simulink library "marine_hydro"  (Simulink 7.4)
settings: Solver=ode45  SolverMode=SingleTasking  StartTime=0.0  StopTime=10.0  RelTol=1e-3
undefined symbols (not defined in the file or in its folder): Hoerner, magnitude, slcm, vessel, vesselABC
libraries: simulink x60, marine_gnc x22, marine_hydro x9
(part 3 of 4)

== system marine_hydro/Hydro Library/Wave loads (U=0)/psi1 ==
  k : Inport  OutDataType=sfix(16)  OutScaling=2^0
  0 or 1 : Inport  Port=2  OutDataType=sfix(16)  OutScaling=2^0
  Gain1 : Gain  Gain=20  ParameterDataType=sfix(16)  ParameterScaling=2^0  OutDataType=sfix(16)  OutScaling=2^0
  Gain2 : Gain  Gain=10  ParameterDataType=sfix(16)  ParameterScaling=2^0  OutDataType=sfix(16)  OutScaling=2^0
  Product : Product  OutDataType=sfix(16)  OutScaling=2^0  RndMeth=Zero
  Sum7 : Sum  Inputs=-+|  OutDataType=sfix(16)  OutScaling=2^0
  Sum8 : Sum  Inputs=++|  OutDataType=sfix(16)  OutScaling=2^0
  const : Constant  Value=18  OutDataType=sfix(16)  OutScaling=2^0
  psi : Outport  OutDataType=sfix(16)  OutScaling=2^0
  wires:
  const/1 -> Sum7/2
  Sum7/1 -> Gain1/1
  Gain1/1 -> Product/1
  Product/1 -> Sum8/2
  Gain2/1 -> Sum8/1
  k/1 -> Sum7/1, Gain2/1
  Sum8/1 -> psi/1
  0 or 1/1 -> Product/2

== system marine_hydro/Hydro Library/Wave loads (U=0)/psi2 ==
  k : Inport  OutDataType=sfix(16)  OutScaling=2^0
  0 or 1 : Inport  Port=2  OutDataType=sfix(16)  OutScaling=2^0
  Gain1 : Gain  Gain=20  ParameterDataType=sfix(16)  ParameterScaling=2^0  OutDataType=sfix(16)  OutScaling=2^0
  Gain2 : Gain  Gain=10  ParameterDataType=sfix(16)  ParameterScaling=2^0  OutDataType=sfix(16)  OutScaling=2^0
  Product : Product  OutDataType=sfix(16)  OutScaling=2^0  RndMeth=Zero
  Sum7 : Sum  Inputs=-+|  OutDataType=sfix(16)  OutScaling=2^0
  Sum8 : Sum  Inputs=++|  OutDataType=sfix(16)  OutScaling=2^0
  const : Constant  Value=18  OutDataType=sfix(16)  OutScaling=2^0
  psi : Outport  OutDataType=sfix(16)  OutScaling=2^0
  wires:
  const/1 -> Sum7/2
  Sum7/1 -> Gain1/1
  Gain1/1 -> Product/1
  Product/1 -> Sum8/2
  Gain2/1 -> Sum8/1
  k/1 -> Sum7/1, Gain2/1
  Sum8/1 -> psi/1
  0 or 1/1 -> Product/2

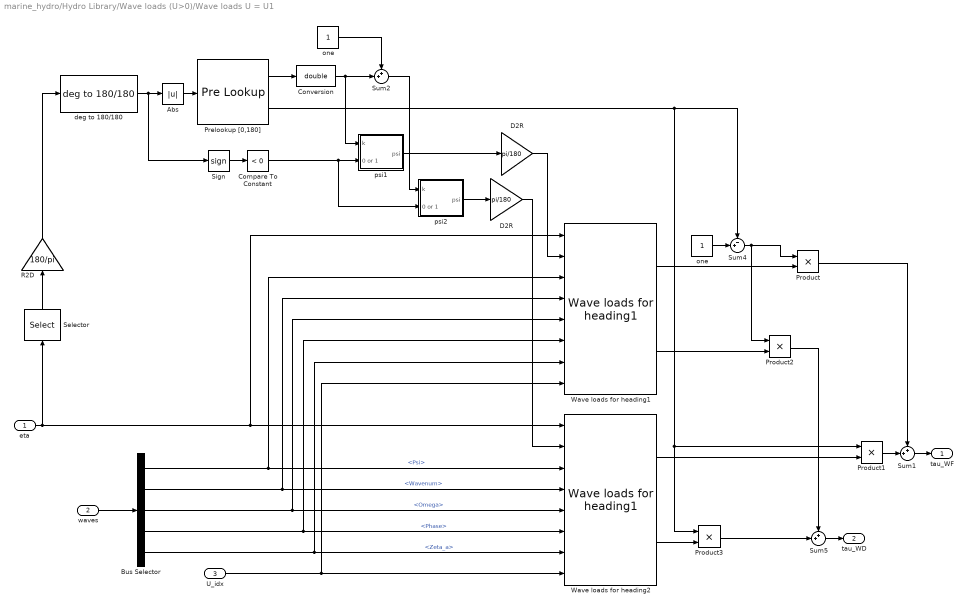
== system marine_hydro/Hydro Library/Wave loads (U>0)/Wave loads U = U1 ==
  eta : Inport  OutDataType=sfix(16)  OutScaling=2^0
  waves : Inport  Port=2  OutDataType=sfix(16)  OutScaling=2^0
  U_idx : Inport  Port=3  OutDataType=sfix(16)  OutScaling=2^0
  Abs : Abs  SaturateOnIntegerOverflow=on
  Bus Selector : BusSelector  OutputSignals=Psi,Wavenum,Omega,Phase,Zeta_a
  Compare To Constant : simulink/Logic and Bit Operations/Compare To Constant  SystemSampleTime=-1  relop=<  const=0  LogicOutDataTypeMode=uint8  ZeroCross=off
  Conversion : DataTypeConversion  OutDataTypeMode=double  OutDataType=sfix(16)  OutScaling=2^0  OutDataTypeStr=double
  D2R : Gain  Gain=pi/180  ParameterDataType=sfix(16)  ParameterScaling=2^0  OutDataType=sfix(16)  OutScaling=2^0
  "D2R " : Gain  Gain=pi/180  ParameterDataType=sfix(16)  ParameterScaling=2^0  OutDataType=sfix(16)  OutScaling=2^0
  Prelookup [0,180] : PreLookup  BreakpointsData=[0:10:180]  IndexSearchMethod=Evenly spaced points  BeginIndexSearchUsingPreviousIndexResult=on  IndexDataType=sfix(16)  FractionDataType=sfix(16)  FractionScaling=2^0
  Product{,1..3} (4 alike) : Product  OutDataType=sfix(16)  OutScaling=2^0  RndMeth=Zero
  R2D : Gain  Gain=180/pi  ParameterDataType=sfix(16)  ParameterScaling=2^0  OutDataType=sfix(16)  OutScaling=2^0
  Selector : Selector  InputPortWidth=6  IndexOptions=Index vector (dialog)  Indices=[6]  OutputSizes=1
  Sign : Signum
  Sum1 : Sum  Inputs=++|  OutDataType=sfix(16)  OutScaling=2^0
  Sum2 : Sum  Inputs=++|  OutDataType=sfix(16)  OutScaling=2^0
  Sum4 : Sum  Inputs=-+|  OutDataType=sfix(16)  OutScaling=2^0
  Sum5 : Sum  Inputs=++|  OutDataType=sfix(16)  OutScaling=2^0
  Wave loads for heading1 : marine_hydro/Hydro Library/Wave loads for heading1  SystemSampleTime=-1  ForceRAO_Freq=vessel.forceRAO.w  WD_Freq=vessel.driftfrc.w  RAO_Vel=vessel.velocities  ForceRAO_Amp=vessel.forceRAO.amp  ForceRAO_Phase=vessel.forceRAO.phase  WD_Amp=vessel.driftfrc.amp  RAO_add_omega_0=on  RAO_add_omega_inf=on
  Wave loads for heading2 : marine_hydro/Hydro Library/Wave loads for heading1  SystemSampleTime=-1  ForceRAO_Freq=vessel.forceRAO.w  WD_Freq=vessel.driftfrc.w  RAO_Vel=vessel.velocities  ForceRAO_Amp=vessel.forceRAO.amp  ForceRAO_Phase=vessel.forceRAO.phase  WD_Amp=vessel.driftfrc.amp  RAO_add_omega_0=on  RAO_add_omega_inf=on
  deg to 180/180 : marine_gnc/Utilities/Math Operations/deg to 180//180  SystemSampleTime=-1
  one : Constant  OutDataType=sfix(16)  OutScaling=2^0
  "one " : Constant  OutDataType=sfix(16)  OutScaling=2^0
  psi1 : Subsystem
  psi2 : Subsystem
  tau_WF : Outport  OutDataType=sfix(16)  OutScaling=2^0
  tau_WD : Outport  Port=2  OutDataType=sfix(16)  OutScaling=2^0
  wires:
  R2D/1 -> deg to 180/180/1
  Selector/1 -> R2D/1
  Sum5/1 -> tau_WD/1
  waves/1 -> Bus Selector/1
  Sum1/1 -> tau_WF/1
  "D2R "/1 -> Wave loads for heading2/2
  D2R/1 -> Wave loads for heading1/2
  psi2/1(psi) -> "D2R "/1
  Conversion/1 -> psi1/1(k), Sum2/2
  Prelookup [0,180]/2 -> Sum4/1, Product1/1, Product3/1
  psi1/1(psi) -> D2R/1
  Compare To Constant/1 -> psi2/2(0 or 1), psi1/2(0 or 1)
  Sign/1 -> Compare To Constant/1
  Abs/1 -> Prelookup [0,180]/1
  deg to 180/180/1 -> Sign/1, Abs/1
  Sum2/1 -> psi2/1(k)
  one/1 -> Sum2/1
  Prelookup [0,180]/1 -> Conversion/1
  Product2/1 -> Sum5/1
  Product3/1 -> Sum5/2
  Wave loads for heading1/2 -> Product2/2
  Sum4/1 -> Product2/1, Product/1
  "one "/1 -> Sum4/2
  Product1/1 -> Sum1/2
  Product/1 -> Sum1/1
  Wave loads for heading1/1 -> Product/2
  Bus Selector/5 -> Wave loads for heading1/7, Wave loads for heading2/7  "<Zeta_a>"
  Bus Selector/4 -> Wave loads for heading1/6, Wave loads for heading2/6  "<Phase>"
  Bus Selector/3 -> Wave loads for heading1/5, Wave loads for heading2/5  "<Omega>"
  Bus Selector/2 -> Wave loads for heading1/4, Wave loads for heading2/4  "<Wavenum>"
  Bus Selector/1 -> Wave loads for heading1/3, Wave loads for heading2/3  "<Psi>"
  eta/1 -> Selector/1, Wave loads for heading1/1, Wave loads for heading2/1
  Wave loads for heading2/2 -> Product3/2
  Wave loads for heading2/1 -> Product1/2
  U_idx/1 -> Wave loads for heading1/8, Wave loads for heading2/8

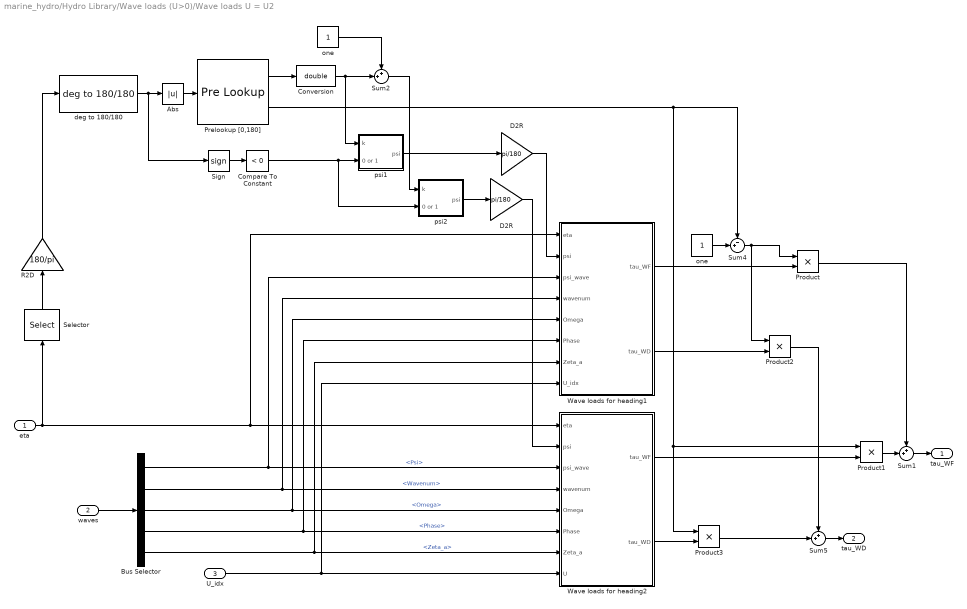
== system marine_hydro/Hydro Library/Wave loads (U>0)/Wave loads U = U2 ==
  eta : Inport  OutDataType=sfix(16)  OutScaling=2^0
  waves : Inport  Port=2  OutDataType=sfix(16)  OutScaling=2^0
  U_idx : Inport  Port=3  OutDataType=sfix(16)  OutScaling=2^0
  Abs : Abs  SaturateOnIntegerOverflow=on
  Bus Selector : BusSelector  OutputSignals=Psi,Wavenum,Omega,Phase,Zeta_a
  Compare To Constant : simulink/Logic and Bit Operations/Compare To Constant  SystemSampleTime=-1  relop=<  const=0  LogicOutDataTypeMode=uint8  ZeroCross=off
  Conversion : DataTypeConversion  OutDataTypeMode=double  OutDataType=sfix(16)  OutScaling=2^0  OutDataTypeStr=double
  D2R : Gain  Gain=pi/180  ParameterDataType=sfix(16)  ParameterScaling=2^0  OutDataType=sfix(16)  OutScaling=2^0
  "D2R " : Gain  Gain=pi/180  ParameterDataType=sfix(16)  ParameterScaling=2^0  OutDataType=sfix(16)  OutScaling=2^0
  Prelookup [0,180] : PreLookup  BreakpointsData=[0:10:180]  IndexSearchMethod=Evenly spaced points  BeginIndexSearchUsingPreviousIndexResult=on  IndexDataType=sfix(16)  FractionDataType=sfix(16)  FractionScaling=2^0
  Product{,1..3} (4 alike) : Product  OutDataType=sfix(16)  OutScaling=2^0  RndMeth=Zero
  R2D : Gain  Gain=180/pi  ParameterDataType=sfix(16)  ParameterScaling=2^0  OutDataType=sfix(16)  OutScaling=2^0
  Selector : Selector  InputPortWidth=6  IndexOptions=Index vector (dialog)  Indices=[6]  OutputSizes=1
  Sign : Signum
  Sum1 : Sum  Inputs=++|  OutDataType=sfix(16)  OutScaling=2^0
  Sum2 : Sum  Inputs=++|  OutDataType=sfix(16)  OutScaling=2^0
  Sum4 : Sum  Inputs=-+|  OutDataType=sfix(16)  OutScaling=2^0
  Sum5 : Sum  Inputs=++|  OutDataType=sfix(16)  OutScaling=2^0
  Wave loads for heading1 : Subsystem  AncestorBlock=marine_gnc/Models/Environmental Loads/Force RAO  mask(Force RAO){ForceRAO_Freq=vessel.forceRAO.w, WD_Freq=vessel.driftfrc.w, RAO_Vel=vessel.velocities, ForceRAO_Amp=vessel.forceRAO.amp, ForceRAO_Phase=vessel.forceRAO.phase, WD_Amp=vessel.driftfrc.amp, RAO_add_omega_0=on, RAO_add_omega_inf=on}
      mask prompts: ForceRAO_Freq "Vector of frequencies ForceRAO_Freq (rad/s)"; WD_Freq "Vector of frequencies WD_Freq (rad/s)"; RAO_Vel "Vector of velocities RAO_Vel (m/s)"; ForceRAO_Amp "6DOF Cell array with tables of Amplitudes ForceRAO_Amp"; ForceRAO_Phase "6DOF Cell array with tables of Phases ForceRAO_Phase (rad)"; WD_Amp "6DOF Cell array with tables of Amplitudes WD_Amp"; RAO_add_omega_0 "Add asymptotic RAO values for omega = 0"; RAO_add_omega_inf "Add asymptotic RAO values for omega = inf"
      mask help:
      | Calculate the 6 degrees-of-freedom (DOF) wave-frequency excitation forces tau_WF for a vessel from its Force Response Amplitude Operators (Force RAOs) and a sea state defined by a set of harmonic waves. The block takes the "Waves" bus from the MSS Waves block as input, as well as the vessel low-frequency (LF) motion in terms of the generalized position vector eta and mean surge velocity U. See help for details.
      |
      | Authors: Oyvind N. Smogeli and Thor I. Fossen, 2005-05-03
      mask init:
      | % use only nonzero increasing velocities, if zero element add eps
      | Nvel = length(RAO_Vel);
      | 
      | if Nvel == 1
      |     RAO_Vel = [0 1e10];   % use one data set for U=0 and one dummy set for u=1e10
      |     Nvel = 2;
      | end
      | 
      | for dof = 1:6
      |     TempFA{dof}  = ForceRAO_Amp{dof}(:,:,1:Nvel);
      |     TempFP{dof}  = ForceRAO_Phase{dof}(:,:,1:Nvel);
      | end
      | 
      | for dof = 1:3
      |     TempWA{dof}  = WD_Amp{dof}(:,:,1:Nvel);
      | end
      | 
      | clear ForceRAO_Amp ForceRAO_Phase WD_Amp WD_Phase
      | 
      | ForceRAO_Amp   = TempFA;
      | ForceRAO_Phase = TempFP;
      | WD_Amp         = TempWA;
      | 
      | % Add RAO values for zero frequency: use values for lowest given frequency
      | if RAO_add_omega_0 > 0
      | 	
      | 	if min(ForceRAO_Freq) > 0
      | 				
      | 		ForceRAO_Freq = [0 ForceRAO_Freq];
      | 		for dofno = 1:6
      | 			ForceRAO_Amp{dofno}   = [ForceRAO_Amp{dofno}(1,:,:);   ForceRAO_Amp{dofno}];
      | 			ForceRAO_Phase{dofno} = [ForceRAO_Phase{dofno}(1,:,:); ForceRAO_Phase{dofno}];
      |         end
      | 
      |     end
      |     
      | 	if min(WD_Freq) > 0
      |         
      | 		WD_Freq = [0 WD_Freq];
      | 		for dofno = 1:3
      | 			WD_Amp{dofno} = [WD_Amp{dofno}(1,:,:); WD_Amp{dofno}];
      | 		end        
      |         
      | 	end
      | 	
      | end
      | 
      | % Add RAO values for high frequency: use values for highest given frequency
      | maxfreq = 10;
      | if RAO_add_omega_inf > 0
      | 
      | 	if max(ForceRAO_Freq) < maxfreq
      | 			
      | 		newfreq = 2*max(ForceRAO_Freq) - ForceRAO_Freq(length(ForceRAO_Freq)-1);
      | 		
      | 		ForceRAO_Freq = [ForceRAO_Freq newfreq maxfreq];
      | 		for dofno = 1:6
      | 			ForceRAO_Amp{dofno}   = [ForceRAO_Amp{dofno};   zeros(2, 36, Nvel)];
      | 			ForceRAO_Phase{dofno} = [ForceRAO_Phase{dofno}; zeros(2, 36, Nvel)];
      | 		end
      | 		
      |     end
      | 
      | 	if max(WD_Freq) < maxfreq
      | 			
      | 		newfreq = 2*max(WD_Freq) - WD_Freq(length(WD_Freq)-1);
      | 		
      | 		WD_Freq = [WD_Freq newfreq maxfreq];
      | 		for dofno = 1:3
      | 			WD_Amp{dofno} = [WD_Amp{dofno}; zeros(2, 36, Nvel)];
      | 		end
      | 		
      |     end
      |     
      | end
      mask Help:
      | <b>Part of the Marine Systems Simulator: MSS</b><br>
      | <br>
      | Calculate the 6 degrees-of-freedom (DOF) wave-frequency excitation forces tau_WF
      | for a vessel from its Force Response Amplitude Operators (Force RAOs) and a sea
      | state defined by a set of harmonic waves. The block takes the &quot;Waves&quot; bus from
      | the MSS Waves block as input, as well as the vessel low-frequency (LF) motion in
      | terms of the generalized position vector eta and mean surge velocity U.<p>The Force RAOs are defined in terms of a
      | vector of frequencies (RAO_Freq), a vector of directions (RAO_Dir), a vector of
      | velocities (RAO_Dir), a 6DOF cell array of 3D matrices with amplitudes
      | (RAO_Amp), and a 6DOF cell array of 3D matrices with phases (RAO_Phase), which
      | are all input in the block mask. The first dimension of the 3D matrices
      | corresponds to the frequencies, the second to the directions, and the third to
      | the velocities, such that e.g. the amplitude amp in heave (DOF #3) for frequency
      | number n_f, direction number n_d and velocity number n_v can be found from a =
      | RAO_Amp{3}(n_f, n_d, n_v).</p>
      | <p><b>Inputs:</b></p>
      | <p>Waves:&nbsp;&nbsp;&nbsp;&nbsp;&nbsp;&nbsp;&nbsp;&nbsp;&nbsp;&nbsp;&nbsp; Bus
      | containing the following signals<br>
      | &nbsp;&nbsp;&nbsp; Zeta_a:&nbsp;&nbsp;&nbsp;&nbsp;&nbsp;&nbsp;&nbsp; Vector of harmonic wave amplitudes [m]<br>
      | &nbsp;&nbsp;&nbsp; Omega:&nbsp;&nbsp;&nbsp;&nbsp;&nbsp;&nbsp; Vector of harmonic wave frequencies [rad/s]<br>
      | &nbsp;&nbsp;&nbsp; Phase:&nbsp;&nbsp;&nbsp;&nbsp;&nbsp;&nbsp;&nbsp;&nbsp; Vector of harmonic wave phases (random) [rad]<br>
      | &nbsp;&nbsp;&nbsp; Wavenum:&nbsp;&nbsp;&nbsp; Vector of harmonic wave numbers [1/m]<br>
      | &nbsp;&nbsp;&nbsp; Psi:&nbsp;&nbsp;&nbsp;&nbsp;&nbsp;&nbsp;&nbsp;&nbsp;&nbsp;&nbsp;&nbsp;&nbsp;&nbsp; Vector of harmonic wave directions [rad]</p>
      | <p>eta_LF:&nbsp;&nbsp;&nbsp;&nbsp;&nbsp;&nbsp;&nbsp;&nbsp;&nbsp;&nbsp;&nbsp;
      | Generalized 6DOF n-frame low-frequency position vector [x (m), y (m), z (m),
      | theta (rad), phi (rad), psi (rad)]<br>
      | U:&nbsp;&nbsp;&nbsp;&nbsp;&nbsp;&nbsp;&nbsp;&nbsp;&nbsp;&nbsp;&nbsp;&nbsp;&nbsp;&nbsp;&nbsp;&nbsp;&nbsp;&nbsp;&nbsp;
      | Low-frequency (mean) surge velocity&nbsp; [m/s]</p>
      | <p><b>Outputs:</b></p>
      | <p>tau_WF:&nbsp;&nbsp;&nbsp;&nbsp;&nbsp;&nbsp;&nbsp;&nbsp;&nbsp; Generalized
      | 6DOF h-frame force vector [X (N), Y (N), Z (N), K (Nm), M (Nm), N (Nm)]</p>
      | <p><b>Model validity:</b></p>
      | <p>The validity of the block is dependent on the validity of the given
      | RAO data set.</p>
      | <p>A proper RAO to be used with this block should contain at least 1 velocity, 5
      | directions (e.g. 0, 45, 90, 135 and 180 degrees) and 10-20 frequencies, for all
      | 6 DOF (surge, sway, heave, roll, pitch, yaw).</p>
      | <p>The block performs linear interpolation in frequencies and directions, and
      | uses the data set for the velocity closest to the input velocity (i.e. 'nearest'
      | interpolation in velocity). If the block recieves an input wave frequency or relative
      | wave direction outside the span of the data vectors RAO_Freq or RAO_Dir
      | respectively, the simulation stops and an error is returned. This means that a well-defined
      | RAO must contain data for both 0 and 180 degrees, and for frequencies covering
      | the desired range of wave frequencies. If desired, asymptotic values can be
      | automatically added for zero and infinity frequency to avoid runtime errors if
      | the wave freqeuncy exceeds the values in RAO_Freq (see checkboxes in the mask). </p>
      | <p>IMPORTANT NOTE: The RAO theory upon which this block is based is in reality
      | only valid when the vessel low-frequency (h-frame) motion is a constant surge
      | velocity only, and the vessel is performing wave-frequency oscillations about
      | the steadily translating h-frame.This means that the outputs from the block when
      | manoeuvering -- i.e. changing the surge velocity and/or yaw angle -- must be
      | interpreted with some care. A jump in the output must be expected when changing
      | between two velocity data sets, and frequency warping expected when changing the
      | yaw angle (due to interpolation in the phase). It is therefore recommended to
      | use backlash on the input velocity to avoid transient switching, and a quantized
      | yaw angle with backlash. The latter will lead to jump in the ouput when the yaw
      | angle changes from one quantized value to another, but will give better results
      | when keeping within one quantizer interval. The quantized yaw angle with
      | backlash and velocity with backlash are available as options via checkboxes in
      | the mask. If either of these are activated, proper values for the yaw
      | quantization interval, yaw backlash width, and the the speed backlash width
      | respectively must be set. Typical values could be a yaw quantization interval of
      | 5 degrees, yaw backlash width of 1/4-1/5 of the quantization interval, and speed
      | backlash width of 1 m/s. To avoid the most rapid transients when switching
      | between data sets, output smoothing is available as an option in the mask. If
      | this is enabled, the output during a transent is rate limited according to the
      | fastest recorded signal rate during normal operation.</p>
      | <p><b>Example mask input:</b></p><p>
      | As an example, the format of the mask input for 2 velocities, 3 directions and 5
      | frequencies is as follows:<p>RAO_Freq = [f1 f2 f3 f4 f5]<br>
      | RAO_Dir = [d1 d2 d3]<br>
      | RAO_Vel = [v1 v2]<p>Surge:<br>
      | RAO_Amp{1}(:,:,1)&nbsp; = [a1_111 a1_121 a1_131; a1_211 a1_221 a1_231; a1_311
      | a1_321 a1_331; a1_411 a1_421 a1_431; a1_511 a1_521 a1_531]<br>
      | RAO_Amp{1}(:,:,2)&nbsp; = [a1_112 a1_122 a1_132; a1_212 a1_222 a1_232; a1_312
      | a1_322 a1_332; a1_412 a1_422 a1_432; a1_512 a1_522 a1_532]<br>
      | RAO_Phase{1}(:,:,1) = [p1_111 p1_121 p1_131; p1_211 p1_221 p1_231; p1_311 p1_321
      | p1_331; p1_411 p1_421 p1_431; p1_511 p1_521 p1_531]<br>
      | RAO_Phase{1}(:,:,2) = [p1_112 p1_122 p1_132; p1_212 p1_222 p1_232; p1_312 p1_322
      | p1_332; p1_412 p1_422 p1_432; p1_512 p1_522 p1_532]<p>Sway:<br>
      | RAO_Amp{2}(:,:,1)&nbsp; = [a2_111 a2_121 a2_131; a2_211 a2_221 a2_231; a2_311
      | a2_321 a2_331; a2_411 a2_421 a2_431; a2_511 a2_521 a2_531]<br>
      | RAO_Amp{2}(:,:,2)&nbsp; = [a2_112 a2_122 a2_132; a2_212 a2_222 a2_232; a2_312
      | a2_322 a2_332; a2_412 a2_422 a2_432; a2_512 a2_522 a2_532]<br>
      | RAO_Phase{2}(:,:,1) = [p2_111 p2_121 p2_131; p2_211 p2_221 p2_231; p2_311 p2_321
      | p2_331; p2_411 p2_421 p2_431; p2_511 p2_521 p2_531]<br>
      | RAO_Phase{2}(:,:,2) = [p2_112 p2_122 p2_132; p2_212 p2_222 p2_232; p2_312 p2_322
      | p2_332; p2_412 p2_422 p2_432; p2_512 p2_522 p2_532]<p>...<p>Yaw:<br>
      | RAO_Amp{6}(:,:,1)&nbsp; = [a6_111 a6_121 a6_131; a6_211 a6_221 a6_231; a6_311
      | a6_321 a6_331; a6_411 a6_421 a6_431; a6_511 a6_521 a6_531]<br>
      | RAO_Amp{6}(:,:,2)&nbsp; = [a6_112 a6_122 a6_132; a6_212 a6_222 a6_232; a6_312
      | a6_322 a6_332; a6_412 a6_422 a6_432; a6_512 a6_522 a6_532]<br>
      | RAO_Phase{6}(:,:,1) = [p6_111 p6_121 p6_131; p6_211 p6_221 p6_231; p6_311 p6_321
      | p6_331; p6_411 p6_421 p6_431; p6_511 p6_521 p6_531]<br>
      | RAO_Phase{6}(:,:,2) = [p6_112 p6_122 p6_132; p6_212 p6_222 p6_232; p6_312 p6_322
      | p6_332; p6_412 p6_422 p6_432; p6_512 p6_522 p6_532]<p>where now for example the
      | amplitude and phase in sway (DOF 2) for frequency f5, direction d3 and velocity
      | v1 are given by RAO_Amp{2}(5,3,1) = a2_531 and RAO_Phase{2}(5,3,1) = p2_531.<p>
      | <b>Copyright (C) NTNU 2005</b></p>
      | <p><b>Author:</b> Oyvind N. Smogeli, 2005-05-03</p>
  Wave loads for heading2 : Subsystem  AncestorBlock=marine_gnc/Models/Environmental Loads/Force RAO  mask(Force RAO){ForceRAO_Freq=vessel.forceRAO.w, WD_Freq=vessel.driftfrc.w, RAO_Vel=vessel.velocities, ForceRAO_Amp=vessel.forceRAO.amp, ForceRAO_Phase=vessel.forceRAO.phase, WD_Amp=vessel.driftfrc.amp, RAO_add_omega_0=on, RAO_add_omega_inf=on}
      mask prompts: ForceRAO_Freq "Vector of frequencies ForceRAO_Freq (rad/s)"; WD_Freq "Vector of frequencies WD_Freq (rad/s)"; RAO_Vel "Vector of velocities RAO_Vel (m/s)"; ForceRAO_Amp "6DOF Cell array with tables of Amplitudes ForceRAO_Amp"; ForceRAO_Phase "6DOF Cell array with tables of Phases ForceRAO_Phase (rad)"; WD_Amp "6DOF Cell array with tables of Amplitudes WD_Amp"; RAO_add_omega_0 "Add asymptotic RAO values for omega = 0"; RAO_add_omega_inf "Add asymptotic RAO values for omega = inf"
      mask help:
      | Calculate the 6 degrees-of-freedom (DOF) wave-frequency excitation forces Tau_WF for a vessel from its Force Response Amplitude Operators (Force RAOs) and a sea state defined by a set of harmonic waves. The block takes the "Waves" bus from the MSS Waves block as input, as well as the vessel low-frequency (LF) motion in terms of the generalized position vector eta_LF and mean surge velocity U. See help for details.
      |
      | Copyright (C) NTNU 2005
      | Author: Oyvind N. Smogeli, 2005-05-03
      mask init: same as marine_hydro/Hydro Library/Wave loads (U>0)/Wave loads U = U2/Wave loads for heading1
      mask Help:
      | <b>Part of the Marine Systems Simulator: MSS</b><br>
      | <br>
      | Calculate the 6 degrees-of-freedom (DOF) wave-frequency excitation forces Tau_WF
      | for a vessel from its Force Response Amplitude Operators (Force RAOs) and a sea
      | state defined by a set of harmonic waves. The block takes the &quot;Waves&quot; bus from
      | the MSS Waves block as input, as well as the vessel low-frequency (LF) motion in
      | terms of the generalized position vector eta_LF and mean surge velocity U.<p>The Force RAOs are defined in terms of a
      | vector of frequencies (RAO_Freq), a vector of directions (RAO_Dir), a vector of
      | velocities (RAO_Dir), a 6DOF cell array of 3D matrices with amplitudes
      | (RAO_Amp), and a 6DOF cell array of 3D matrices with phases (RAO_Phase), which
      | are all input in the block mask. The first dimension of the 3D matrices
      | corresponds to the frequencies, the second to the directions, and the third to
      | the velocities, such that e.g. the amplitude amp in heave (DOF #3) for frequency
      | number n_f, direction number n_d and velocity number n_v can be found from a =
      | RAO_Amp{3}(n_f, n_d, n_v).</p>
      | <p><b>Inputs:</b></p>
      | <p>Waves:&nbsp;&nbsp;&nbsp;&nbsp;&nbsp;&nbsp;&nbsp;&nbsp;&nbsp;&nbsp;&nbsp; Bus
      | containing the following signals<br>
      | &nbsp;&nbsp;&nbsp; Zeta_a:&nbsp;&nbsp;&nbsp;&nbsp;&nbsp;&nbsp;&nbsp; Vector of harmonic wave amplitudes [m]<br>
      | &nbsp;&nbsp;&nbsp; Omega:&nbsp;&nbsp;&nbsp;&nbsp;&nbsp;&nbsp; Vector of harmonic wave frequencies [rad/s]<br>
      | &nbsp;&nbsp;&nbsp; Phase:&nbsp;&nbsp;&nbsp;&nbsp;&nbsp;&nbsp;&nbsp;&nbsp; Vector of harmonic wave phases (random) [rad]<br>
      | &nbsp;&nbsp;&nbsp; Wavenum:&nbsp;&nbsp;&nbsp; Vector of harmonic wave numbers [1/m]<br>
      | &nbsp;&nbsp;&nbsp; Psi:&nbsp;&nbsp;&nbsp;&nbsp;&nbsp;&nbsp;&nbsp;&nbsp;&nbsp;&nbsp;&nbsp;&nbsp;&nbsp; Vector of harmonic wave directions [rad]</p>
      | <p>eta_LF:&nbsp;&nbsp;&nbsp;&nbsp;&nbsp;&nbsp;&nbsp;&nbsp;&nbsp;&nbsp;&nbsp;
      | Generalized 6DOF n-frame low-frequency position vector [x (m), y (m), z (m),
      | theta (rad), phi (rad), psi (rad)]<br>
      | U:&nbsp;&nbsp;&nbsp;&nbsp;&nbsp;&nbsp;&nbsp;&nbsp;&nbsp;&nbsp;&nbsp;&nbsp;&nbsp;&nbsp;&nbsp;&nbsp;&nbsp;&nbsp;&nbsp;
      | Low-frequency (mean) surge velocity&nbsp; [m/s]</p>
      | <p><b>Outputs:</b></p>
      | <p>tau_WF:&nbsp;&nbsp;&nbsp;&nbsp;&nbsp;&nbsp;&nbsp;&nbsp;&nbsp; Generalized
      | 6DOF h-frame force vector [X (N), Y (N), Z (N), K (Nm), M (Nm), N (Nm)]</p>
      | <p><b>Model validity:</b></p>
      | <p>The validity of the block is dependent on the validity of the given
      | RAO data set.</p>
      | <p>A proper RAO to be used with this block should contain at least 1 velocity, 5
      | directions (e.g. 0, 45, 90, 135 and 180 degrees) and 10-20 frequencies, for all
      | 6 DOF (surge, sway, heave, roll, pitch, yaw).</p>
      | <p>The block performs linear interpolation in frequencies and directions, and
      | uses the data set for the velocity closest to the input velocity (i.e. 'nearest'
      | interpolation in velocity). If the block recieves an input wave frequency or relative
      | wave direction outside the span of the data vectors RAO_Freq or RAO_Dir
      | respectively, the simulation stops and an error is returned. This means that a well-defined
      | RAO must contain data for both 0 and 180 degrees, and for frequencies covering
      | the desired range of wave frequencies. If desired, asymptotic values can be
      | automatically added for zero and infinity frequency to avoid runtime errors if
      | the wave freqeuncy exceeds the values in RAO_Freq (see checkboxes in the mask). </p>
      | <p>IMPORTANT NOTE: The RAO theory upon which this block is based is in reality
      | only valid when the vessel low-frequency (h-frame) motion is a constant surge
      | velocity only, and the vessel is performing wave-frequency oscillations about
      | the steadily translating h-frame.This means that the outputs from the block when
      | manoeuvering -- i.e. changing the surge velocity and/or yaw angle -- must be
      | interpreted with some care. A jump in the output must be expected when changing
      | between two velocity data sets, and frequency warping expected when changing the
      | yaw angle (due to interpolation in the phase). It is therefore recommended to
      | use backlash on the input velocity to avoid transient switching, and a quantized
      | yaw angle with backlash. The latter will lead to jump in the ouput when the yaw
      | angle changes from one quantized value to another, but will give better results
      | when keeping within one quantizer interval. The quantized yaw angle with
      | backlash and velocity with backlash are available as options via checkboxes in
      | the mask. If either of these are activated, proper values for the yaw
      | quantization interval, yaw backlash width, and the the speed backlash width
      | respectively must be set. Typical values could be a yaw quantization interval of
      | 5 degrees, yaw backlash width of 1/4-1/5 of the quantization interval, and speed
      | backlash width of 1 m/s. To avoid the most rapid transients when switching
      | between data sets, output smoothing is available as an option in the mask. If
      | this is enabled, the output during a transent is rate limited according to the
      | fastest recorded signal rate during normal operation.</p>
      | <p><b>Example mask input:</b></p><p>
      | As an example, the format of the mask input for 2 velocities, 3 directions and 5
      | frequencies is as follows:<p>RAO_Freq = [f1 f2 f3 f4 f5]<br>
      | RAO_Dir = [d1 d2 d3]<br>
      | RAO_Vel = [v1 v2]<p>Surge:<br>
      | RAO_Amp{1}(:,:,1)&nbsp; = [a1_111 a1_121 a1_131; a1_211 a1_221 a1_231; a1_311
      | a1_321 a1_331; a1_411 a1_421 a1_431; a1_511 a1_521 a1_531]<br>
      | RAO_Amp{1}(:,:,2)&nbsp; = [a1_112 a1_122 a1_132; a1_212 a1_222 a1_232; a1_312
      | a1_322 a1_332; a1_412 a1_422 a1_432; a1_512 a1_522 a1_532]<br>
      | RAO_Phase{1}(:,:,1) = [p1_111 p1_121 p1_131; p1_211 p1_221 p1_231; p1_311 p1_321
      | p1_331; p1_411 p1_421 p1_431; p1_511 p1_521 p1_531]<br>
      | RAO_Phase{1}(:,:,2) = [p1_112 p1_122 p1_132; p1_212 p1_222 p1_232; p1_312 p1_322
      | p1_332; p1_412 p1_422 p1_432; p1_512 p1_522 p1_532]<p>Sway:<br>
      | RAO_Amp{2}(:,:,1)&nbsp; = [a2_111 a2_121 a2_131; a2_211 a2_221 a2_231; a2_311
      | a2_321 a2_331; a2_411 a2_421 a2_431; a2_511 a2_521 a2_531]<br>
      | RAO_Amp{2}(:,:,2)&nbsp; = [a2_112 a2_122 a2_132; a2_212 a2_222 a2_232; a2_312
      | a2_322 a2_332; a2_412 a2_422 a2_432; a2_512 a2_522 a2_532]<br>
      | RAO_Phase{2}(:,:,1) = [p2_111 p2_121 p2_131; p2_211 p2_221 p2_231; p2_311 p2_321
      | p2_331; p2_411 p2_421 p2_431; p2_511 p2_521 p2_531]<br>
      | RAO_Phase{2}(:,:,2) = [p2_112 p2_122 p2_132; p2_212 p2_222 p2_232; p2_312 p2_322
      | p2_332; p2_412 p2_422 p2_432; p2_512 p2_522 p2_532]<p>...<p>Yaw:<br>
      | RAO_Amp{6}(:,:,1)&nbsp; = [a6_111 a6_121 a6_131; a6_211 a6_221 a6_231; a6_311
      | a6_321 a6_331; a6_411 a6_421 a6_431; a6_511 a6_521 a6_531]<br>
      | RAO_Amp{6}(:,:,2)&nbsp; = [a6_112 a6_122 a6_132; a6_212 a6_222 a6_232; a6_312
      | a6_322 a6_332; a6_412 a6_422 a6_432; a6_512 a6_522 a6_532]<br>
      | RAO_Phase{6}(:,:,1) = [p6_111 p6_121 p6_131; p6_211 p6_221 p6_231; p6_311 p6_321
      | p6_331; p6_411 p6_421 p6_431; p6_511 p6_521 p6_531]<br>
      | RAO_Phase{6}(:,:,2) = [p6_112 p6_122 p6_132; p6_212 p6_222 p6_232; p6_312 p6_322
      | p6_332; p6_412 p6_422 p6_432; p6_512 p6_522 p6_532]<p>where now for example the
      | amplitude and phase in sway (DOF 2) for frequency f5, direction d3 and velocity
      | v1 are given by RAO_Amp{2}(5,3,1) = a2_531 and RAO_Phase{2}(5,3,1) = p2_531.<p>
      | <b>Copyright (C) NTNU 2005</b></p>
      | <p><b>Author:</b> Oyvind N. Smogeli, 2005-05-03</p>
  deg to 180/180 : marine_gnc/Utilities/Math Operations/deg to 180//180  SystemSampleTime=-1
  one : Constant  OutDataType=sfix(16)  OutScaling=2^0
  "one " : Constant  OutDataType=sfix(16)  OutScaling=2^0
  psi1 : Subsystem
  psi2 : Subsystem
  tau_WF : Outport  OutDataType=sfix(16)  OutScaling=2^0
  tau_WD : Outport  Port=2  OutDataType=sfix(16)  OutScaling=2^0
  wires:
  R2D/1 -> deg to 180/180/1
  Selector/1 -> R2D/1
  Sum5/1 -> tau_WD/1
  waves/1 -> Bus Selector/1
  Sum1/1 -> tau_WF/1
  "D2R "/1 -> Wave loads for heading2/2(psi)
  D2R/1 -> Wave loads for heading1/2(psi)
  psi2/1(psi) -> "D2R "/1
  Conversion/1 -> psi1/1(k), Sum2/2
  Prelookup [0,180]/2 -> Sum4/1, Product1/1, Product3/1
  psi1/1(psi) -> D2R/1
  Compare To Constant/1 -> psi2/2(0 or 1), psi1/2(0 or 1)
  Sign/1 -> Compare To Constant/1
  Abs/1 -> Prelookup [0,180]/1
  deg to 180/180/1 -> Sign/1, Abs/1
  Sum2/1 -> psi2/1(k)
  one/1 -> Sum2/1
  Prelookup [0,180]/1 -> Conversion/1
  Product2/1 -> Sum5/1
  Product3/1 -> Sum5/2
  Wave loads for heading1/2(tau_WD) -> Product2/2
  Sum4/1 -> Product2/1, Product/1
  "one "/1 -> Sum4/2
  Product1/1 -> Sum1/2
  Product/1 -> Sum1/1
  Wave loads for heading1/1(tau_WF) -> Product/2
  Bus Selector/5 -> Wave loads for heading2/7(Zeta_a), Wave loads for heading1/7(Zeta_a)  "<Zeta_a>"
  Bus Selector/4 -> Wave loads for heading2/6(Phase), Wave loads for heading1/6(Phase)  "<Phase>"
  Bus Selector/3 -> Wave loads for heading2/5(Omega), Wave loads for heading1/5(Omega)  "<Omega>"
  Bus Selector/2 -> Wave loads for heading2/4(wavenum), Wave loads for heading1/4(wavenum)  "<Wavenum>"
  Bus Selector/1 -> Wave loads for heading2/3(psi_wave), Wave loads for heading1/3(psi_wave)  "<Psi>"
  eta/1 -> Selector/1, Wave loads for heading1/1(eta), Wave loads for heading2/1(eta)
  Wave loads for heading2/2(tau_WD) -> Product3/2
  Wave loads for heading2/1(tau_WF) -> Product1/2
  U_idx/1 -> Wave loads for heading2/8(U), Wave loads for heading1/8(U_idx)

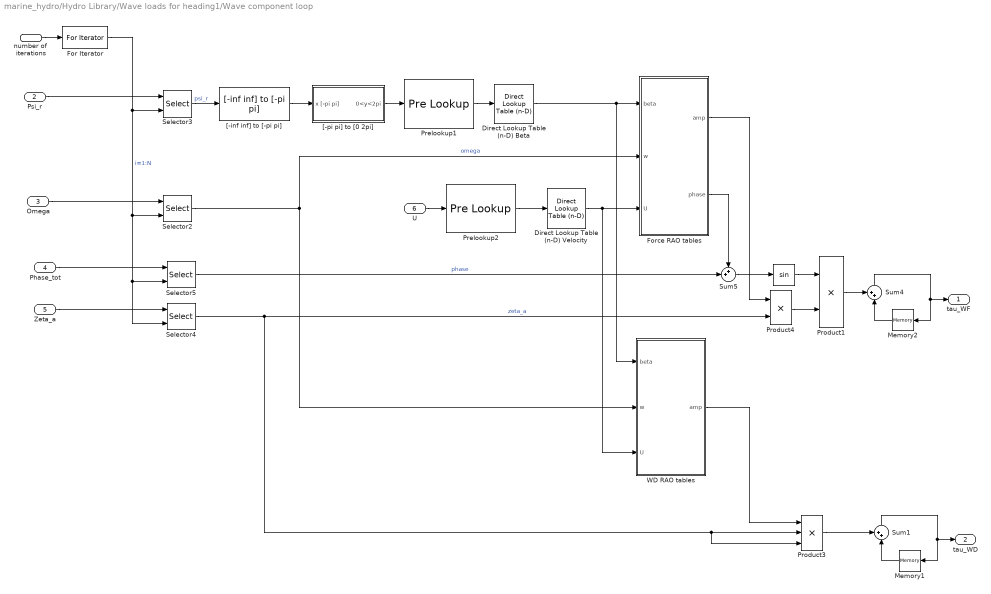
== system marine_hydro/Hydro Library/Wave loads for heading1/Wave component loop ==
  number of  iterations : Inport  OutDataType=sfix(16)  OutScaling=2^0
  Psi_r : Inport  Port=2  OutDataType=sfix(16)  OutScaling=2^0
  Omega : Inport  Port=3  OutDataType=sfix(16)  OutScaling=2^0
  Phase_tot : Inport  Port=4  OutDataType=sfix(16)  OutScaling=2^0
  Zeta_a : Inport  Port=5  OutDataType=sfix(16)  OutScaling=2^0
  U : Inport  Port=6  OutDataType=sfix(16)  OutScaling=2^0
  "                " : Trigonometry
  Direct Lookup Table (n-D) Beta : simulink/Lookup Tables/Direct Lookup Table (n-D)  maskTabDims=1  explicitNumDims=1  outDims=Element  tabIsInput=off  mxTable=vessel.headings  clipFlag=Warning  samptime=-1
  Direct Lookup Table (n-D) Velocity : simulink/Lookup Tables/Direct Lookup Table (n-D)  maskTabDims=1  explicitNumDims=1  outDims=Element  tabIsInput=off  mxTable=RAO_Vel  clipFlag=Warning  samptime=-1
  For Iterator : ForIterator  ResetStates=reset  IterationSource=external  IterationVariableDataType=double
  Force RAO tables : Subsystem
      mask Type: RAO table lookup
      mask Description:
      | Perform 3D table lookup in 6DOF RAO amplitudes and phases, using the relative wave heading psi_r, wave frequency omega and vessel velocity vel as inputs. See documentation of the Motion RAO block or Force RAO block for details. A warning is issued if the input is outside the range spanned by the RAOs.
      | 
      | Author: Oyvind N. Smogeli and Thor I. Fossen, 2005-05-03
  Memory1 : Memory  X0=[0 0 0 0 0 0]'  InheritSampleTime=on
  Memory2 : Memory  X0=[0 0 0 0 0 0]'  InheritSampleTime=on
  Prelookup1 : PreLookup  BreakpointsData=vessel.headings  IndexSearchMethod=Evenly spaced points  BeginIndexSearchUsingPreviousIndexResult=on  OutputOnlyTheIndex=on  IndexDataType=sfix(16)  FractionDataType=sfix(16)  FractionScaling=2^0
  Prelookup2 : PreLookup  BreakpointsData=RAO_Vel  IndexSearchMethod=Linear search  BeginIndexSearchUsingPreviousIndexResult=on  OutputOnlyTheIndex=on  IndexDataType=sfix(16)  FractionDataType=sfix(16)  FractionScaling=2^0
  Product1 : Product  OutDataType=sfix(16)  OutScaling=2^0  SaturateOnIntegerOverflow=on  OutDataTypeStr=Inherit: Same as first input
  Product3 : Product  Inputs=3  OutDataType=sfix(16)  OutScaling=2^0  SaturateOnIntegerOverflow=on  OutDataTypeStr=Inherit: Same as first input
  Product4 : Product  OutDataType=sfix(16)  OutScaling=2^0  SaturateOnIntegerOverflow=on  OutDataTypeStr=Inherit: Same as first input
  Selector{2..5} (4 alike) : Selector  IndexOptions=Index vector (port)  Indices=[1 3]  OutputSizes=1
  Sum1 : Sum  Inputs=++|  OutDataType=sfix(16)  OutScaling=2^0  SaturateOnIntegerOverflow=on
  Sum4 : Sum  Inputs=++|  OutDataType=sfix(16)  OutScaling=2^0  SaturateOnIntegerOverflow=on
  Sum5 : Sum  Inputs=++|  OutDataType=sfix(16)  OutScaling=2^0  SaturateOnIntegerOverflow=on
  WD RAO tables : Subsystem
      mask Type: RAO table lookup
      mask Description:
      | Perform 3D table lookup in 6DOF RAO amplitudes and phases, using the relative wave heading psi_r, wave frequency omega and vessel velocity vel as inputs. See documentation of the Motion RAO block or Force RAO block for details. A warning is issued if the input is outside the range spanned by the RAOs.
      | 
      | Author: Oyvind N. Smogeli and Thor I. Fossen, 2005-05-03
  "[-inf inf] to [-pi pi]" : marine_gnc/Utilities/Math Operations/[-inf inf] to [-pi pi]  SystemSampleTime=-1
  "[-pi pi] to [0 2pi]" : Subsystem
      mask Type: [-inf inf] to [-pi pi]
      mask Description: Converts an angle in rad to (-pi pi)
  tau_WF : Outport  OutDataType=sfix(16)  OutScaling=2^0
  tau_WD : Outport  Port=2  OutDataType=sfix(16)  OutScaling=2^0
  wires:
  Selector4/1 -> Product4/2, Product3/2, Product3/3  "zeta_a"
  Sum5/1 -> "                "/1
  Zeta_a/1 -> Selector4/1
  Phase_tot/1 -> Selector5/1
  U/1 -> Prelookup2/1
  Psi_r/1 -> Selector3/1
  Omega/1 -> Selector2/1
  number of  iterations/1 -> For Iterator/1
  Sum4/1 -> Memory2/1, tau_WF/1
  Memory2/1 -> Sum4/2
  Product1/1 -> Sum4/1
  Selector5/1 -> Sum5/2  "phase"
  Selector3/1 -> "[-inf inf] to [-pi pi]"/1  "psi_r"
  "                "/1 -> Product1/1
  Product4/1 -> Product1/2
  Sum1/1 -> Memory1/1, tau_WD/1
  Memory1/1 -> Sum1/2
  Product3/1 -> Sum1/1
  "[-pi pi] to [0 2pi]"/1(0<y<2pi) -> Prelookup1/1
  Selector2/1 -> Force RAO tables/2(w), WD RAO tables/2(w)  "omega"
  For Iterator/1 -> Selector3/2, Selector2/2, Selector4/2, Selector5/2  "i=1:N"
  "[-inf inf] to [-pi pi]"/1 -> "[-pi pi] to [0 2pi]"/1(x [-pi pi])
  Prelookup1/1 -> Direct Lookup Table (n-D) Beta/1
  Direct Lookup Table (n-D) Beta/1 -> Force RAO tables/1(beta), WD RAO tables/1(beta)
  Prelookup2/1 -> Direct Lookup Table (n-D) Velocity/1
  Direct Lookup Table (n-D) Velocity/1 -> Force RAO tables/3(U), WD RAO tables/3(U)
  Force RAO tables/2(phase) -> Sum5/1
  Force RAO tables/1(amp) -> Product4/1
  WD RAO tables/1(amp) -> Product3/1

== system marine_hydro/Hydro Library/6 DOF DP model  (zero speed model with fluid memory)/Fluid memory effetcs/heave ==
  nu : Inport  OutDataType=sfix(16)  OutScaling=2^0
  Selector : Selector  InputPortWidth=6  IndexOptions=Index vector (dialog)  Indices=[1]  OutputSizes=1
  Selector1 : Selector  InputPortWidth=6  IndexOptions=Index vector (dialog)  Indices=[3]  OutputSizes=1
  Selector2 : Selector  InputPortWidth=6  IndexOptions=Index vector (dialog)  Indices=[5]  OutputSizes=1
  u : Outport  OutDataType=sfix(16)  OutScaling=2^0
  w : Outport  Port=2  OutDataType=sfix(16)  OutScaling=2^0
  q : Outport  Port=3  OutDataType=sfix(16)  OutScaling=2^0
  wires:
  nu/1 -> Selector/1, Selector1/1, Selector2/1
  Selector/1 -> u/1
  Selector1/1 -> w/1
  Selector2/1 -> q/1

== system marine_hydro/Hydro Library/6 DOF DP model  (zero speed model with fluid memory)/Fluid memory effetcs/pitch ==
  nu : Inport  OutDataType=sfix(16)  OutScaling=2^0
  Selector : Selector  InputPortWidth=6  IndexOptions=Index vector (dialog)  Indices=[1]  OutputSizes=1
  Selector1 : Selector  InputPortWidth=6  IndexOptions=Index vector (dialog)  Indices=[3]  OutputSizes=1
  Selector2 : Selector  InputPortWidth=6  IndexOptions=Index vector (dialog)  Indices=[5]  OutputSizes=1
  u : Outport  OutDataType=sfix(16)  OutScaling=2^0
  w : Outport  Port=2  OutDataType=sfix(16)  OutScaling=2^0
  q : Outport  Port=3  OutDataType=sfix(16)  OutScaling=2^0
  wires:
  nu/1 -> Selector/1, Selector1/1, Selector2/1
  Selector/1 -> u/1
  Selector1/1 -> w/1
  Selector2/1 -> q/1

== system marine_hydro/Hydro Library/6 DOF DP model  (zero speed model with fluid memory)/Fluid memory effetcs/roll ==
  nu : Inport  OutDataType=sfix(16)  OutScaling=2^0
  Selector : Selector  InputPortWidth=6  IndexOptions=Index vector (dialog)  Indices=[2]  OutputSizes=1
  Selector1 : Selector  InputPortWidth=6  IndexOptions=Index vector (dialog)  Indices=[4]  OutputSizes=1
  Selector2 : Selector  InputPortWidth=6  IndexOptions=Index vector (dialog)  Indices=[6]  OutputSizes=1
  v : Outport  OutDataType=sfix(16)  OutScaling=2^0
  p : Outport  Port=2  OutDataType=sfix(16)  OutScaling=2^0
  r : Outport  Port=3  OutDataType=sfix(16)  OutScaling=2^0
  wires:
  nu/1 -> Selector/1, Selector1/1, Selector2/1
  Selector/1 -> v/1
  Selector1/1 -> p/1
  Selector2/1 -> r/1

== system marine_hydro/Hydro Library/6 DOF DP model  (zero speed model with fluid memory)/Fluid memory effetcs/surge ==
  nu : Inport  OutDataType=sfix(16)  OutScaling=2^0
  Selector : Selector  InputPortWidth=6  IndexOptions=Index vector (dialog)  Indices=[1]  OutputSizes=1
  Selector1 : Selector  InputPortWidth=6  IndexOptions=Index vector (dialog)  Indices=[3]  OutputSizes=1
  Selector2 : Selector  InputPortWidth=6  IndexOptions=Index vector (dialog)  Indices=[5]  OutputSizes=1
  u : Outport  OutDataType=sfix(16)  OutScaling=2^0
  w : Outport  Port=2  OutDataType=sfix(16)  OutScaling=2^0
  q : Outport  Port=3  OutDataType=sfix(16)  OutScaling=2^0
  wires:
  nu/1 -> Selector/1, Selector1/1, Selector2/1
  Selector/1 -> u/1
  Selector1/1 -> w/1
  Selector2/1 -> q/1

== system marine_hydro/Hydro Library/6 DOF DP model  (zero speed model with fluid memory)/Fluid memory effetcs/sway ==
  nu : Inport  OutDataType=sfix(16)  OutScaling=2^0
  Selector : Selector  InputPortWidth=6  IndexOptions=Index vector (dialog)  Indices=[2]  OutputSizes=1
  Selector1 : Selector  InputPortWidth=6  IndexOptions=Index vector (dialog)  Indices=[4]  OutputSizes=1
  Selector2 : Selector  InputPortWidth=6  IndexOptions=Index vector (dialog)  Indices=[6]  OutputSizes=1
  v : Outport  OutDataType=sfix(16)  OutScaling=2^0
  p : Outport  Port=2  OutDataType=sfix(16)  OutScaling=2^0
  r : Outport  Port=3  OutDataType=sfix(16)  OutScaling=2^0
  wires:
  nu/1 -> Selector/1, Selector1/1, Selector2/1
  Selector/1 -> v/1
  Selector1/1 -> p/1
  Selector2/1 -> r/1

== system marine_hydro/Hydro Library/6 DOF DP model  (zero speed model with fluid memory)/Fluid memory effetcs/yaw ==
  nu : Inport  OutDataType=sfix(16)  OutScaling=2^0
  Selector : Selector  InputPortWidth=6  IndexOptions=Index vector (dialog)  Indices=[2]  OutputSizes=1
  Selector1 : Selector  InputPortWidth=6  IndexOptions=Index vector (dialog)  Indices=[4]  OutputSizes=1
  Selector2 : Selector  InputPortWidth=6  IndexOptions=Index vector (dialog)  Indices=[6]  OutputSizes=1
  v : Outport  OutDataType=sfix(16)  OutScaling=2^0
  p : Outport  Port=2  OutDataType=sfix(16)  OutScaling=2^0
  r : Outport  Port=3  OutDataType=sfix(16)  OutScaling=2^0
  wires:
  nu/1 -> Selector/1, Selector1/1, Selector2/1
  Selector/1 -> v/1
  Selector1/1 -> p/1
  Selector2/1 -> r/1

== system marine_hydro/Hydro Library/6 DOF Maneuvering model  (unified model with fluid memory)/Fluid memory effetcs/heave ==
  nu : Inport  OutDataType=sfix(16)  OutScaling=2^0
  Selector : Selector  InputPortWidth=6  IndexOptions=Index vector (dialog)  Indices=[1]  OutputSizes=1
  Selector1 : Selector  InputPortWidth=6  IndexOptions=Index vector (dialog)  Indices=[3]  OutputSizes=1
  Selector2 : Selector  InputPortWidth=6  IndexOptions=Index vector (dialog)  Indices=[5]  OutputSizes=1
  u : Outport  OutDataType=sfix(16)  OutScaling=2^0
  w : Outport  Port=2  OutDataType=sfix(16)  OutScaling=2^0
  q : Outport  Port=3  OutDataType=sfix(16)  OutScaling=2^0
  wires:
  nu/1 -> Selector/1, Selector1/1, Selector2/1
  Selector/1 -> u/1
  Selector1/1 -> w/1
  Selector2/1 -> q/1

== system marine_hydro/Hydro Library/6 DOF Maneuvering model  (unified model with fluid memory)/Fluid memory effetcs/pitch ==
  nu : Inport  OutDataType=sfix(16)  OutScaling=2^0
  Selector : Selector  InputPortWidth=6  IndexOptions=Index vector (dialog)  Indices=[1]  OutputSizes=1
  Selector1 : Selector  InputPortWidth=6  IndexOptions=Index vector (dialog)  Indices=[3]  OutputSizes=1
  Selector2 : Selector  InputPortWidth=6  IndexOptions=Index vector (dialog)  Indices=[5]  OutputSizes=1
  u : Outport  OutDataType=sfix(16)  OutScaling=2^0
  w : Outport  Port=2  OutDataType=sfix(16)  OutScaling=2^0
  q : Outport  Port=3  OutDataType=sfix(16)  OutScaling=2^0
  wires:
  nu/1 -> Selector/1, Selector1/1, Selector2/1
  Selector/1 -> u/1
  Selector1/1 -> w/1
  Selector2/1 -> q/1

== system marine_hydro/Hydro Library/6 DOF Maneuvering model  (unified model with fluid memory)/Fluid memory effetcs/roll ==
  nu : Inport  OutDataType=sfix(16)  OutScaling=2^0
  Selector : Selector  InputPortWidth=6  IndexOptions=Index vector (dialog)  Indices=[2]  OutputSizes=1
  Selector1 : Selector  InputPortWidth=6  IndexOptions=Index vector (dialog)  Indices=[4]  OutputSizes=1
  Selector2 : Selector  InputPortWidth=6  IndexOptions=Index vector (dialog)  Indices=[6]  OutputSizes=1
  v : Outport  OutDataType=sfix(16)  OutScaling=2^0
  p : Outport  Port=2  OutDataType=sfix(16)  OutScaling=2^0
  r : Outport  Port=3  OutDataType=sfix(16)  OutScaling=2^0
  wires:
  nu/1 -> Selector/1, Selector1/1, Selector2/1
  Selector/1 -> v/1
  Selector1/1 -> p/1
  Selector2/1 -> r/1

== system marine_hydro/Hydro Library/6 DOF Maneuvering model  (unified model with fluid memory)/Fluid memory effetcs/surge ==
  nu : Inport  OutDataType=sfix(16)  OutScaling=2^0
  Selector : Selector  InputPortWidth=6  IndexOptions=Index vector (dialog)  Indices=[1]  OutputSizes=1
  Selector1 : Selector  InputPortWidth=6  IndexOptions=Index vector (dialog)  Indices=[3]  OutputSizes=1
  Selector2 : Selector  InputPortWidth=6  IndexOptions=Index vector (dialog)  Indices=[5]  OutputSizes=1
  u : Outport  OutDataType=sfix(16)  OutScaling=2^0
  w : Outport  Port=2  OutDataType=sfix(16)  OutScaling=2^0
  q : Outport  Port=3  OutDataType=sfix(16)  OutScaling=2^0
  wires:
  nu/1 -> Selector/1, Selector1/1, Selector2/1
  Selector/1 -> u/1
  Selector1/1 -> w/1
  Selector2/1 -> q/1

== system marine_hydro/Hydro Library/6 DOF Maneuvering model  (unified model with fluid memory)/Fluid memory effetcs/sway ==
  nu : Inport  OutDataType=sfix(16)  OutScaling=2^0
  Selector : Selector  InputPortWidth=6  IndexOptions=Index vector (dialog)  Indices=[2]  OutputSizes=1
  Selector1 : Selector  InputPortWidth=6  IndexOptions=Index vector (dialog)  Indices=[4]  OutputSizes=1
  Selector2 : Selector  InputPortWidth=6  IndexOptions=Index vector (dialog)  Indices=[6]  OutputSizes=1
  v : Outport  OutDataType=sfix(16)  OutScaling=2^0
  p : Outport  Port=2  OutDataType=sfix(16)  OutScaling=2^0
  r : Outport  Port=3  OutDataType=sfix(16)  OutScaling=2^0
  wires:
  nu/1 -> Selector/1, Selector1/1, Selector2/1
  Selector/1 -> v/1
  Selector1/1 -> p/1
  Selector2/1 -> r/1

== system marine_hydro/Hydro Library/6 DOF Maneuvering model  (unified model with fluid memory)/Fluid memory effetcs/yaw ==
  nu : Inport  OutDataType=sfix(16)  OutScaling=2^0
  Selector : Selector  InputPortWidth=6  IndexOptions=Index vector (dialog)  Indices=[2]  OutputSizes=1
  Selector1 : Selector  InputPortWidth=6  IndexOptions=Index vector (dialog)  Indices=[4]  OutputSizes=1
  Selector2 : Selector  InputPortWidth=6  IndexOptions=Index vector (dialog)  Indices=[6]  OutputSizes=1
  v : Outport  OutDataType=sfix(16)  OutScaling=2^0
  p : Outport  Port=2  OutDataType=sfix(16)  OutScaling=2^0
  r : Outport  Port=3  OutDataType=sfix(16)  OutScaling=2^0
  wires:
  nu/1 -> Selector/1, Selector1/1, Selector2/1
  Selector/1 -> v/1
  Selector1/1 -> p/1
  Selector2/1 -> r/1

== system marine_hydro/Hydro Library/6 DOF Maneuvering model  (unified model with fluid memory)/Model Info1/EmptySubsystem ==

== system marine_hydro/Hydro Library/Cross-flow drag and surge resistance/Cross-flow drag trapezoidal integration/multiply with 0.5 ==
  In1 : Inport  OutDataType=sfix(16)  OutScaling=2^0
  Action Port : ActionPort  InitializeStates=reset
  Gain : Gain  Gain=0.5  ParameterDataType=sfix(16)  ParameterScaling=2^0  OutDataType=sfix(16)  OutScaling=2^0
  Out1 : Outport  OutDataType=sfix(16)  OutScaling=2^0
  wires:
  Gain/1 -> Out1/1
  In1/1 -> Gain/1

== system marine_hydro/Hydro Library/Cross-flow drag and surge resistance/Cross-flow drag trapezoidal integration/multiply with 1 ==
  In1 : Inport  OutDataType=sfix(16)  OutScaling=2^0
  Action Port : ActionPort  InitializeStates=reset
  Out1 : Outport  OutDataType=sfix(16)  OutScaling=2^0
  wires:
  In1/1 -> Out1/1

== system marine_hydro/Hydro Library/WD for heading1/Wave component loop/WD RAO tables ==
  beta : Inport  OutDataType=sfix(16)  OutScaling=2^0
  w : Inport  Port=2  OutDataType=sfix(16)  OutScaling=2^0
  U : Inport  Port=3  OutDataType=sfix(16)  OutScaling=2^0
  Constant : Constant  Value=0  OutDataType=sfix(16)  OutScaling=2^0
  Lookup Table (n-D)  Wavedrift 1 : simulink/Lookup Tables/Lookup Table (n-D)  numDimsPopupSelect=3  bp1=WD_Freq  bp2=vessel.headings  bp3=RAO_Vel  bp4=[1:3]  bpcell={ [1:3], [1:3] }  explicitNumDims=2  searchMode=Linear Search  cacheBpFlag=on  vectorInputFlag=off  tableData=WD_Amp{1}  interpMethod=Linear  extrapMethod=None - Clip  rangeErrorMode=Warning
  Lookup Table (n-D)  Wavedrift 2 : simulink/Lookup Tables/Lookup Table (n-D)  numDimsPopupSelect=3  bp1=WD_Freq  bp2=vessel.headings  bp3=RAO_Vel  bp4=[1:3]  bpcell={ [1:3], [1:3] }  explicitNumDims=2  searchMode=Linear Search  cacheBpFlag=on  vectorInputFlag=off  tableData=WD_Amp{2}  interpMethod=Linear  extrapMethod=None - Clip  rangeErrorMode=Warning
  Lookup Table (n-D)  Wavedrift 3 : simulink/Lookup Tables/Lookup Table (n-D)  numDimsPopupSelect=3  bp1=WD_Freq  bp2=vessel.headings  bp3=RAO_Vel  bp4=[1:3]  bpcell={ [1:3], [1:3] }  explicitNumDims=2  searchMode=Linear Search  cacheBpFlag=on  vectorInputFlag=off  tableData=WD_Amp{3}  interpMethod=Linear  extrapMethod=None - Clip  rangeErrorMode=Warning
  Mux1 : Mux  Inputs=6
  amp : Outport  OutDataType=sfix(16)  OutScaling=2^0
  wires:
  w/1 -> Lookup Table (n-D)  Wavedrift 1/1, Lookup Table (n-D)  Wavedrift 3/1, Lookup Table (n-D)  Wavedrift 2/1
  Constant/1 -> Mux1/5, Mux1/4, Mux1/3
  beta/1 -> Lookup Table (n-D)  Wavedrift 1/2, Lookup Table (n-D)  Wavedrift 3/2, Lookup Table (n-D)  Wavedrift 2/2
  U/1 -> Lookup Table (n-D)  Wavedrift 1/3, Lookup Table (n-D)  Wavedrift 3/3, Lookup Table (n-D)  Wavedrift 2/3
  Lookup Table (n-D)  Wavedrift 1/1 -> Mux1/1
  Lookup Table (n-D)  Wavedrift 2/1 -> Mux1/2
  Lookup Table (n-D)  Wavedrift 3/1 -> Mux1/6
  Mux1/1 -> amp/1

== system marine_hydro/Hydro Library/WD for heading1/Wave component loop/[-pi pi] to [0 2pi] ==
  note: x
  x [-pi pi] : Inport  OutDataType=sfix(16)  OutScaling=2^0
  Constant : Constant  Value=2*pi  OutDataType=sfix(16)  OutScaling=2^0
  Constant1 : Constant  Value=0  OutDataType=sfix(16)  OutScaling=2^0
  Sign : Signum
  Sum : Sum  Inputs=|++  OutDataType=sfix(16)  OutScaling=2^0  SaturateOnIntegerOverflow=on
  Switch : Switch
  0<y<2pi : Outport  OutDataType=sfix(16)  OutScaling=2^0
  wires:
  Constant1/1 -> Switch/1
  Constant/1 -> Switch/3
  Sign/1 -> Switch/2
  Sum/1 -> 0<y<2pi/1
  Switch/1 -> Sum/1
  x [-pi pi]/1 -> Sum/2, Sign/1

== system marine_hydro/Hydro Library/Wave loads (U>0)/Wave loads U = U1/psi1 ==
  k : Inport  OutDataType=sfix(16)  OutScaling=2^0
  0 or 1 : Inport  Port=2  OutDataType=sfix(16)  OutScaling=2^0
  Gain1 : Gain  Gain=20  ParameterDataType=sfix(16)  ParameterScaling=2^0  OutDataType=sfix(16)  OutScaling=2^0
  Gain2 : Gain  Gain=10  ParameterDataType=sfix(16)  ParameterScaling=2^0  OutDataType=sfix(16)  OutScaling=2^0
  Product : Product  OutDataType=sfix(16)  OutScaling=2^0  RndMeth=Zero
  Sum7 : Sum  Inputs=-+|  OutDataType=sfix(16)  OutScaling=2^0
  Sum8 : Sum  Inputs=++|  OutDataType=sfix(16)  OutScaling=2^0
  const : Constant  Value=18  OutDataType=sfix(16)  OutScaling=2^0
  psi : Outport  OutDataType=sfix(16)  OutScaling=2^0
  wires:
  0 or 1/1 -> Product/2
  Sum8/1 -> psi/1
  k/1 -> Gain2/1, Sum7/1
  Gain2/1 -> Sum8/1
  Product/1 -> Sum8/2
  Gain1/1 -> Product/1
  Sum7/1 -> Gain1/1
  const/1 -> Sum7/2
